simulink model "PID"  (R2024a)
settings: Solver=VariableStepAuto  StartTime=0.0  StopTime=12  RelTol=1e-3
settings Model: Creator=thunguyen  LastModifiedBy=thunguyen

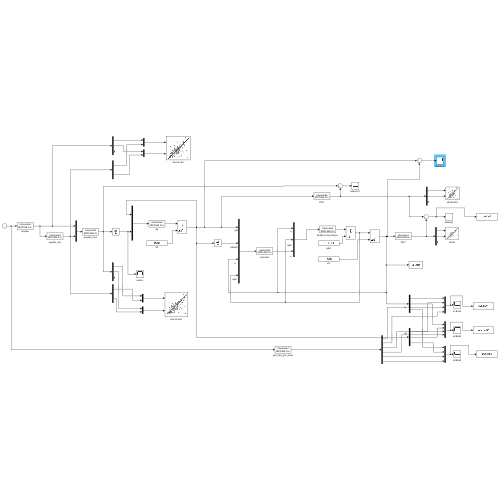
[thumbnail: Simulink's stored preview of the top-level diagram]
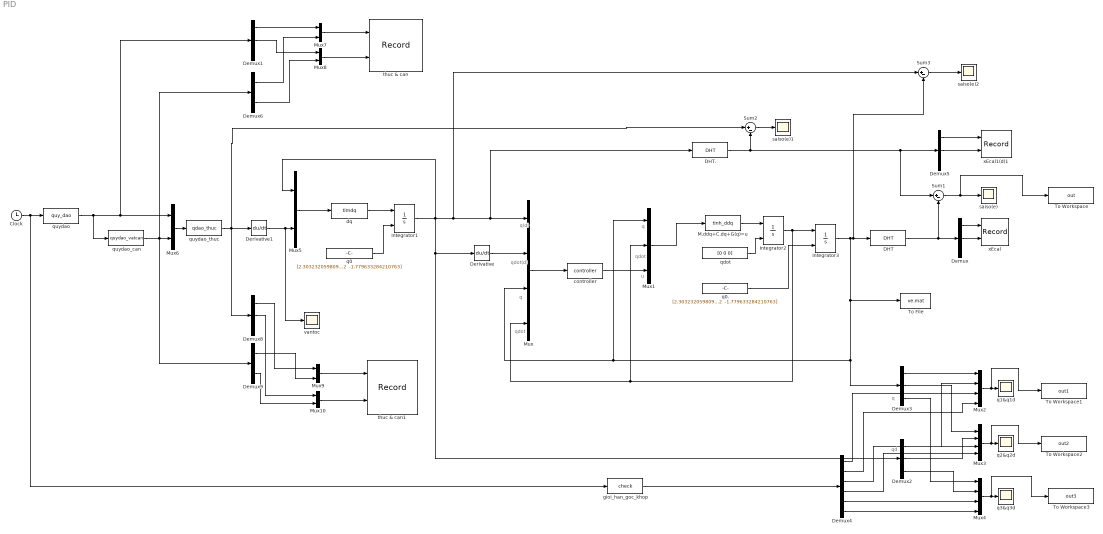
== system PID ==
  note: qd
  note: q
  note: u
  note: qdot
  note: qdot(d)
  note: q
  note: q
  note: q(d)
  note: qdot
  Clock : Clock
      settings: Decimation=2
  DHT : MATLABFcn  MATLABFcn=DHT  OutputDimensions=3  Output1D=off
  DHT. : MATLABFcn  MATLABFcn=DHT  OutputDimensions=3  Output1D=off
  Demux{,1..3,5,8} (6 alike) : Demux  Outputs=3
  Demux4 : Demux  Outputs=6
  Demux6 : Demux  Outputs=2
  Demux9 : Demux  Outputs=2
  Derivative : Derivative
  Derivative1 : Derivative
  Integrator1 : Integrator  InitialConditionSource=external  InitialCondition=1
  Integrator2 : Integrator  InitialConditionSource=external  InitialCondition=1
  Integrator3 : Integrator  InitialConditionSource=external  InitialCondition=1
  M.ddq+C.dq+G(q)=u : MATLABFcn  MATLABFcn=tinh_ddq  OutputDimensions=3  Output1D=off
  Mux{,2..4} (4 alike) : Mux
  Mux1 : Mux  Inputs=3
  Mux{5..10} (6 alike) : Mux  Inputs=2
  Sum1 : Sum  Inputs=|+-
  Sum2 : Sum  Inputs=|+-
  Sum3 : Sum  Inputs=|+-
  To File : ToFile  Filename=ve.mat
  To Workspace : ToWorkspace  VariableName=out  SaveFormat=Timeseries  SampleTime=-1
  To Workspace1 : ToWorkspace  VariableName=out1  SaveFormat=Timeseries  SampleTime=-1
  To Workspace2 : ToWorkspace  VariableName=out2  SaveFormat=Timeseries  SampleTime=-1
  To Workspace3 : ToWorkspace  VariableName=out3  SaveFormat=Timeseries  SampleTime=-1
  controller : MATLABFcn  MATLABFcn=controller  OutputDimensions=3  Output1D=off
  dq : MATLABFcn  MATLABFcn=timdq  OutputDimensions=3  Output1D=off
  gioi_han_goc_khop : MATLABFcn  MATLABFcn=check  OutputDimensions=6
  q0 : Constant  Value="[2.303232059809062   0.120492197697522  -1.779633284210763]"  VectorParams1D=off
  q0. : Constant  Value="[2.303232059809062   0.120492197697522  -1.779633284210763]"  VectorParams1D=off
  q1&q1d : Scope
  q2&q2d : Scope
  q3&q3d : Scope
  qdot : Constant  Value=[0 0 0]  VectorParams1D=off
  quydao : MATLABFcn  MATLABFcn=quy_dao  OutputDimensions=3
  quydao_can : MATLABFcn  MATLABFcn=quydao_vatcan  OutputDimensions=2
  quydao_thuc : MATLABFcn  MATLABFcn=qdao_thuc  OutputDimensions=3
  saiso(e) : Scope
  saiso(e)1 : Scope
  saiso(e)2 : Scope
  thuc & can : Record  FileSettingsInternal="{\"entries\":[{\"content\":{\"excelSettings\":{\"content\":{},\"type\":\"Streamout.ExcelSettings\"}},\"type\":\"Streamout.FileSettingStorage\",\"uuid\":\"\"}],\"packageUris\":[\"http:\\/\\/schema.mathworks.com\\/mf0\\/streamout_blocks\\/R2020a\"],\"version\":\"1.0\"}"  Layout=[1 1]  SignalsInternal="{\"entries\":[{\"content\":{\"signals\":[{\"content\":{\"blockPath\":[],\"dimensions\":[2],\"domain\":\"\",\"hasChildren\":true,\"lineColor\":\"#a2142f\",\"lineWidth\":2,\"port\":1,\"sid\":[\"\"],\"signalID\":1,\"signalName\":\"Mux7\"},\"type\":\"RecordBlkView.Signal\",\"uuid\":\"\"},{\"content\":{\"blockPath\":[],\"channel\":[1],\"dimensions\":[2],\"domain\":\"\",\"lineColor\":\"#b746ff\",\"lineWidth\":2,\"parentID\":1,\"plots\":[ 1 ],\"port\":1,\"sid\":[\"\"],\"signalID\":2,\"signalName\":\"Mux7\"},\"type\":\"RecordBlkView.Signal\",\"uuid\":\"\"},{\"content\":{\"blockPath\":[],\"dimensions\":[2],\"domain\":\"\",\"hasChildren\":true,\"lineColor\":\"#ff6929\",\"lineWidth\":2,\"port\":2,\"sid\":[\"\"],\"signalID\":3,\"signalName\":\"Mux8\"},\"type\":\"RecordBlkView.Signal\",\"uuid\":\"\"},{\"content\":{\"blockPath\":[],\"channel\":[1],\"dimensions\":[2],\"domain\":\"\",\"lineColor\":\"#ff13a6\",\"lineWidth\":2,\"parentID\":3,\"plots\":[ 1 ],\"port\":2,\"sid\":[\"\"],\"signalID\":4,\"signalName\":\"Mux8\"},\"type\":\"RecordBlkView.Signal\",\"uuid\":\"\"},{\"content\":{\"blockPath\":[],\"channel\":[2],\"dimensions\":[2],\"domain\":\"\",\"lineColor\":\"#ff6929\",\"lineWidth\":2,\"parentID\":1,\"plots\":[ 1 ],\"port\":1,\"sid\":[\"\"],\"signalID\":5,\"signalName\":\"Mux7\"},\"type\":\"RecordBlkView.Signal\",\"uuid\":\"\"},{\"content\":{\"blockPath\":[],\"channel\":[2],\"dimensions\":[2],\"domain\":\"\",\"lineColor\":\"#b746ff\",\"lineWidth\":2,\"parentID\":3,\"plots\":[ 1 ],\"port\":2,\"sid\":[\"\"],\"signalID\":6,\"signalName\":\"Mux8\"},\"type\":\"RecordBlkView.Signal\",\"uuid\":\"\"}]},\"type\":\"RecordBlkView.InputSignals\",\"uuid\":\"\"}],\"packageUris\":[\"http:\\/\\/schema.mathworks.com\\/mf0\\/streamout_blocks\\/R2020a\"],\"version\":\"1.0\"}"  VisualizationBindings="{\"xyplotplugin\":{\"info\":[{\"series\":[{\"bindingParametersList\":[{\"parameter\":\"X-Axis\",\"signalID\":2,\"signalName\":\"Mux7(1)\"},{\"parameter\":\"Y-Axis\",\"signalID\":4,\"signalName\":\"Mux8(1)\"}],\"seriesID\":0},{\"bindingParametersList\":[{\"parameter\":\"X-Axis\",\"signalID\":5,\"signalName\":\"Mux7(2)\"},{\"parameter\":\"Y-Axis\",\"signalID\":6,\"signalName\":\"Mux8(2)\"}],\"seriesID\":1}],\"subplotID\":1}]}}"  CompatibilityTag=XY
  thuc & can1 : Record  FileSettingsInternal="{\"entries\":[{\"content\":{\"excelSettings\":{\"content\":{},\"type\":\"Streamout.ExcelSettings\"}},\"type\":\"Streamout.FileSettingStorage\",\"uuid\":\"\"}],\"packageUris\":[\"http:\\/\\/schema.mathworks.com\\/mf0\\/streamout_blocks\\/R2020a\"],\"version\":\"1.0\"}"  Layout=[1 1]  SignalsInternal="{\"entries\":[{\"content\":{\"signals\":[{\"content\":{\"blockPath\":[],\"dimensions\":[2],\"domain\":\"\",\"hasChildren\":true,\"lineColor\":\"#64d413\",\"lineWidth\":2,\"port\":1,\"sid\":[\"\"],\"signalID\":1,\"signalName\":\"Mux9\"},\"type\":\"RecordBlkView.Signal\",\"uuid\":\"\"},{\"content\":{\"blockPath\":[],\"channel\":[1],\"dimensions\":[2],\"domain\":\"\",\"lineColor\":\"#b746ff\",\"lineWidth\":2,\"parentID\":1,\"plots\":[ 1 ],\"port\":1,\"sid\":[\"\"],\"signalID\":2,\"signalName\":\"Mux9\"},\"type\":\"RecordBlkView.Signal\",\"uuid\":\"\"},{\"content\":{\"blockPath\":[],\"dimensions\":[2],\"domain\":\"\",\"hasChildren\":true,\"lineColor\":\"#fe330a\",\"lineWidth\":2,\"port\":2,\"sid\":[\"\"],\"signalID\":3,\"signalName\":\"Mux10\"},\"type\":\"RecordBlkView.Signal\",\"uuid\":\"\"},{\"content\":{\"blockPath\":[],\"channel\":[1],\"dimensions\":[2],\"domain\":\"\",\"lineColor\":\"#ff13a6\",\"lineWidth\":2,\"parentID\":3,\"plots\":[ 1 ],\"port\":2,\"sid\":[\"\"],\"signalID\":4,\"signalName\":\"Mux10\"},\"type\":\"RecordBlkView.Signal\",\"uuid\":\"\"},{\"content\":{\"blockPath\":[],\"channel\":[2],\"dimensions\":[2],\"domain\":\"\",\"lineColor\":\"#fe330a\",\"lineWidth\":2,\"parentID\":1,\"plots\":[ 1 ],\"port\":1,\"sid\":[\"\"],\"signalID\":5,\"signalName\":\"Mux9\"},\"type\":\"RecordBlkView.Signal\",\"uuid\":\"\"},{\"content\":{\"blockPath\":[],\"channel\":[2],\"dimensions\":[2],\"domain\":\"\",\"lineColor\":\"#22b573\",\"lineWidth\":2,\"parentID\":3,\"plots\":[ 1 ],\"port\":2,\"sid\":[\"\"],\"signalID\":6,\"signalName\":\"Mux10\"},\"type\":\"RecordBlkView.Signal\",\"uuid\":\"\"}]},\"type\":\"RecordBlkView.InputSignals\",\"uuid\":\"\"}],\"packageUris\":[\"http:\\/\\/schema.mathworks.com\\/mf0\\/streamout_blocks\\/R2020a\"],\"version\":\"1.0\"}"  VisualizationBindings="{\"xyplotplugin\":{\"info\":[{\"series\":[{\"bindingParametersList\":[{\"parameter\":\"X-Axis\",\"signalID\":2,\"signalName\":\"Mux9(1)\"},{\"parameter\":\"Y-Axis\",\"signalID\":4,\"signalName\":\"Mux10(1)\"}],\"seriesID\":0},{\"bindingParametersList\":[{\"parameter\":\"X-Axis\",\"signalID\":5,\"signalName\":\"Mux9(2)\"},{\"parameter\":\"Y-Axis\",\"signalID\":6,\"signalName\":\"Mux10(2)\"}],\"seriesID\":1}],\"subplotID\":1}]}}"  CompatibilityTag=XY
  vantoc : Scope
  xEcal : Record  FileSettingsInternal="{\"entries\":[{\"content\":{\"excelSettings\":{\"content\":{},\"type\":\"Streamout.ExcelSettings\"}},\"type\":\"Streamout.FileSettingStorage\",\"uuid\":\"\"}],\"packageUris\":[\"http:\\/\\/schema.mathworks.com\\/mf0\\/streamout_blocks\\/R2020a\"],\"version\":\"1.0\"}"  Layout=[1 1]  SignalsInternal="{\"entries\":[{\"content\":{\"signals\":[{\"content\":{\"blockPath\":[],\"dimensions\":[1],\"domain\":\"\",\"lineColor\":\"#edb120\",\"lineWidth\":2,\"plots\":[ 1 ],\"port\":1,\"sid\":[\"\"],\"signalID\":1,\"signalName\":\"Demux:1\"},\"type\":\"RecordBlkView.Signal\",\"uuid\":\"\"},{\"content\":{\"blockPath\":[],\"dimensions\":[1],\"domain\":\"\",\"lineColor\":\"#7e2f8e\",\"lineWidth\":2,\"plots\":[ 1 ],\"port\":2,\"sid\":[\"\"],\"signalID\":2,\"signalName\":\"Demux:2\"},\"type\":\"RecordBlkView.Signal\",\"uuid\":\"\"}]},\"type\":\"RecordBlkView.InputSignals\",\"uuid\":\"\"}],\"packageUris\":[\"http:\\/\\/schema.mathworks.com\\/mf0\\/streamout_blocks\\/R2020a\"],\"version\":\"1.0\"}"  VisualizationBindings="{\"xyplotplugin\":{\"info\":[{\"series\":[{\"bindingParametersList\":[{\"parameter\":\"X-Axis\",\"signalID\":1,\"signalName\":\"Demux:1\"},{\"parameter\":\"Y-Axis\",\"signalID\":2,\"signalName\":\"Demux:2\"}],\"seriesID\":0}],\"subplotID\":1}]}}"  CompatibilityTag=XY
  xEcal1(d)1 : Record  FileSettingsInternal="{\"entries\":[{\"content\":{\"excelSettings\":{\"content\":{},\"type\":\"Streamout.ExcelSettings\"}},\"type\":\"Streamout.FileSettingStorage\",\"uuid\":\"\"}],\"packageUris\":[\"http:\\/\\/schema.mathworks.com\\/mf0\\/streamout_blocks\\/R2020a\"],\"version\":\"1.0\"}"  Layout=[1 1]  SignalsInternal="{\"entries\":[{\"content\":{\"signals\":[{\"content\":{\"blockPath\":[],\"dimensions\":[1],\"domain\":\"\",\"lineColor\":\"#fe330a\",\"lineWidth\":2,\"plots\":[ 1 ],\"port\":1,\"sid\":[\"\"],\"signalID\":1,\"signalName\":\"Demux5:1\"},\"type\":\"RecordBlkView.Signal\",\"uuid\":\"\"},{\"content\":{\"blockPath\":[],\"dimensions\":[1],\"domain\":\"\",\"lineColor\":\"#22b573\",\"lineWidth\":2,\"plots\":[ 1 ],\"port\":2,\"sid\":[\"\"],\"signalID\":2,\"signalName\":\"Demux5:2\"},\"type\":\"RecordBlkView.Signal\",\"uuid\":\"\"}]},\"type\":\"RecordBlkView.InputSignals\",\"uuid\":\"\"}],\"packageUris\":[\"http:\\/\\/schema.mathworks.com\\/mf0\\/streamout_blocks\\/R2020a\"],\"version\":\"1.0\"}"  VisualizationBindings="{\"xyplotplugin\":{\"info\":[{\"series\":[{\"bindingParametersList\":[{\"parameter\":\"X-Axis\",\"signalID\":1,\"signalName\":\"Demux5:1\"},{\"parameter\":\"Y-Axis\",\"signalID\":2,\"signalName\":\"Demux5:2\"}],\"seriesID\":0}],\"subplotID\":1}]}}"  CompatibilityTag=XY
  wires:
  Clock/1 -> quydao/1, gioi_han_goc_khop/1
  DHT/1 -> Sum1/2, Demux/1
  Demux/1 -> xEcal/1
  Demux/2 -> xEcal/2
  M.ddq+C.dq+G(q)=u/1 -> Integrator2/1
  Integrator2/1 -> Mux/4, Mux1/2, Integrator3/1
  qdot/1 -> Integrator2/2
  Sum1/1 -> To Workspace/1, saiso(e)/1
  Mux/1 -> controller/1
  Mux1/1 -> M.ddq+C.dq+G(q)=u/1
  controller/1 -> Mux1/3
  Integrator3/1 -> Sum3/2, DHT/1, Demux3/1, Mux1/1, Mux/3, To File/1
  Mux2/1 -> To Workspace1/1, q1&q1d/1
  Mux4/1 -> To Workspace3/1, q3&q3d/1
  Mux3/1 -> To Workspace2/1, q2&q2d/1
  Demux3/1 -> Mux2/1
  Demux2/1 -> Mux2/2
  Demux3/2 -> Mux3/1
  Demux2/2 -> Mux3/2
  Demux3/3 -> Mux4/1
  Demux2/3 -> Mux4/2
  Derivative/1 -> Mux/2
  Mux5/1 -> dq/1
  dq/1 -> Integrator1/1
  Integrator1/1 -> Demux2/1, Derivative/1, Mux5/1, Sum3/1, DHT./1, Mux/1
  gioi_han_goc_khop/1 -> Demux4/1
  Demux4/1 -> Mux2/3
  Demux4/2 -> Mux2/4
  Demux4/3 -> Mux3/3
  Demux4/4 -> Mux3/4
  Demux4/5 -> Mux4/3
  Demux4/6 -> Mux4/4
  q0./1 -> Integrator3/2
  q0/1 -> Integrator1/2
  Demux5/1 -> xEcal1(d)1/1
  Demux5/2 -> xEcal1(d)1/2
  quydao/1 -> Demux1/1, Mux6/1, quydao_can/1
  Derivative1/1 -> vantoc/1, Mux5/2
  Mux6/1 -> quydao_thuc/1
  Demux1/2 -> Mux8/1
  Demux1/1 -> Mux7/1
  Mux7/1 -> thuc & can/1
  Mux8/1 -> thuc & can/2
  Demux6/1 -> Mux7/2
  Demux6/2 -> Mux8/2
  Demux9/1 -> Mux9/2
  Mux10/1 -> thuc & can1/2
  Demux9/2 -> Mux10/2
  Mux9/1 -> thuc & can1/1
  quydao_can/1 -> Mux6/2, Demux6/1, Demux9/1
  Demux8/1 -> Mux9/1
  Demux8/2 -> Mux10/1
  Sum2/1 -> saiso(e)1/1
  quydao_thuc/1 -> Sum2/1, Derivative1/1, Demux8/1
  DHT./1 -> Sum1/1, Demux5/1, Sum2/2
  Sum3/1 -> saiso(e)2/1
